simulink model "model_maglev"  (R2024a)
settings: Solver=VariableStepAuto  StartTime=0.0  StopTime=10.0  RelTol=1e-3
undefined symbols (not defined in the file): A, Cd, ci, fiP1, fiP2, g, ki, m, R, rho, v0, z0
settings Model: Creator=Bocchio  LastModifiedBy=Bocchio

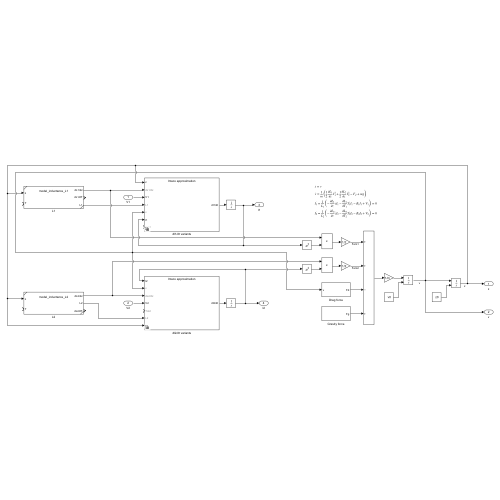
[thumbnail: Simulink's stored preview of the top-level diagram]
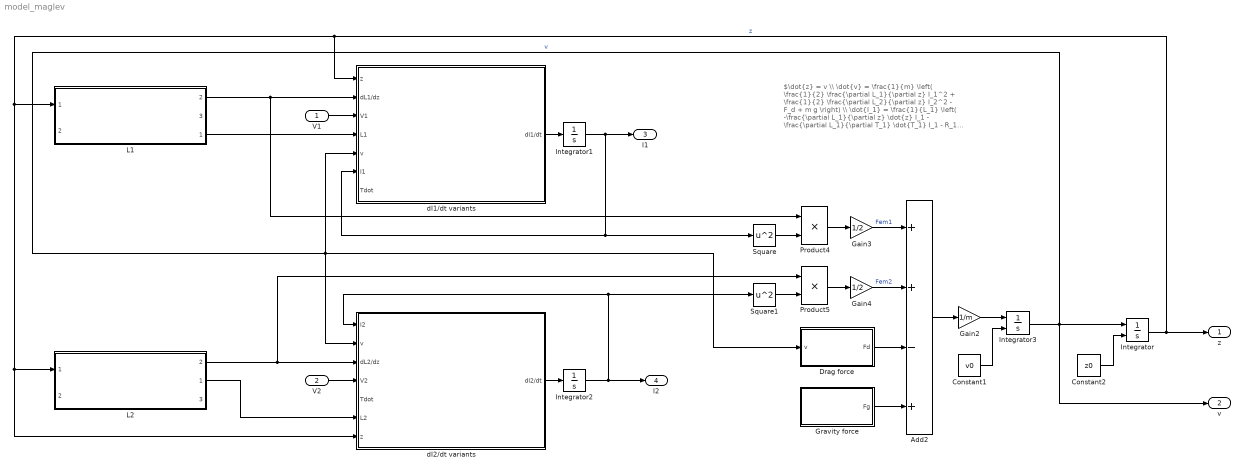
== system model_maglev ==
  note: $\dot{z} = v \\ \dot{v} = \frac{1}{m} \left( \frac{1}{2} \frac{\partial L_1}{\partial z} I_1^2 + \frac{1}{2} \frac{\partial L_2}{\partial z} I_2^2 - F_d + m g \right) \\ \dot{I_1} = \frac{1}{L_1} \left( -\frac{\partial L_1}{\partial z} \dot{z} I_1 - \frac{\partial L_1}{\partial T_1} \dot{T_1} I_1 - R_1 I_1 + V_1 \right) = 0 \\ \dot{I_2} = \frac{1}{L_2} \left( -\frac{\partial L_2}{\partial z} \dot{z} I_2 - \frac{\partial L_2}{\partial T_2} \dot{T_2} I_2 - R_2 I_2 + V_2 \right) = 0$
  V1 : Inport
  V2 : Inport  Port=2
  Add2 : Sum  Inputs=++-+
  Constant1 : Constant  Value=v0
  Constant2 : Constant  Value=z0
  Drag force : Subsystem
  Gain2 : Gain  Gain=1/m
  Gain3 : Gain  Gain=1/2
  Gain4 : Gain  Gain=1/2
  Gravity force : Subsystem
  Integrator : Integrator  InitialConditionSource=external
  Integrator1 : Integrator
  Integrator2 : Integrator
  Integrator3 : Integrator  InitialConditionSource=external
  L1 : Subsystem  ReferencedSubsystem=model_inductance_L1
      settings: PortSchema="{\"entries\":[{\"content\":{\"sides\":[{\"content\":{\"connectorIds\":[\"In1\",\"In2\"]},\"type\":\"ConnectorPlacement.EquallySpacedRectSide\",\"uuid\":\"7eb98e79-1222-4180-ad1b-16015b2454e9\"},{\"content\":{\"connectorIds\":[\"Out2\",\"Out3\",\"Out1\"],\"side\":\"RIGHT\"},\"type\":\"ConnectorPlacement.EquallySpacedRectSide\",\"uuid\":\"ce7d8014-b2ab-4313-9aa1-af3c9ff32da8\"},{\"content\":{\"side\":\"TOP\"},\"type\":\"ConnectorPlacement.EquallySpacedRectSide\",\"uuid\":\"6bd72466-ab25-4d86-adcd-22d1f13a01c9\"}]},\"type\":\"ConnectorPlacement.EquallySpacedConnector\",\"uuid\":\"baaaeab3-d8cd-49b4-9261-57480d9625ca\"}],\"packageUris\":[\"http://schema.mathworks.com/mf0/Connector/R2020b\"],\"version\":\"1.0\"}"
  L2 : Subsystem  ReferencedSubsystem=model_inductance_L2
      settings: PortSchema="{\"entries\":[{\"content\":{\"sides\":[{\"content\":{\"connectorIds\":[\"In1\",\"In2\"]},\"type\":\"ConnectorPlacement.EquallySpacedRectSide\",\"uuid\":\"1e02beb1-2eb2-4867-b71d-7851c60b3d68\"},{\"content\":{\"connectorIds\":[\"Out2\",\"Out1\",\"Out3\"],\"side\":\"RIGHT\"},\"type\":\"ConnectorPlacement.EquallySpacedRectSide\",\"uuid\":\"344f63f1-a805-4e14-b05f-49edc1fe2f4c\"},{\"content\":{\"side\":\"TOP\"},\"type\":\"ConnectorPlacement.EquallySpacedRectSide\",\"uuid\":\"d9945970-5ec1-4fd6-a2b8-3934b3c2782b\"}]},\"type\":\"ConnectorPlacement.EquallySpacedConnector\",\"uuid\":\"87b64261-f50a-433f-9b00-8a3b81ee7894\"}],\"packageUris\":[\"http://schema.mathworks.com/mf0/Connector/R2020b\"],\"version\":\"1.0\"}"
  Product4 : Product
  Product5 : Product
  Square : Math  Operator=square
  Square1 : Math  Operator=square
  dI1/dt variants : Subsystem  Variant=on  VariantControlMode=label  LabelModeActiveChoice=false
  dI2/dt variants : Subsystem  Variant=on  VariantControlMode=label  LabelModeActiveChoice=false
  z : Outport
  v : Outport  Port=2
  I1 : Outport  Port=3
  I2 : Outport  Port=4
  wires:
  Integrator/1 -> z/1, dI2/dt variants/7(z), L2/1, L1/1, dI1/dt variants/1(z)  "z"
  L1/1 -> dI1/dt variants/4(L1)
  Gain3/1 -> Add2/1  "Fem1"
  L2/1 -> dI2/dt variants/6(L2)
  dI1/dt variants/1(dI1/dt) -> Integrator1/1
  Gain4/1 -> Add2/2  "Fem2"
  Square/1 -> Product4/2
  Square1/1 -> Product5/2
  Integrator1/1 -> Square/1, dI1/dt variants/6(I1), I1/1
  Add2/1 -> Gain2/1
  Product4/1 -> Gain3/1
  Product5/1 -> Gain4/1
  Integrator3/1 -> v/1, Drag force/1(v), dI2/dt variants/2(v), dI1/dt variants/5(v), Integrator/1  "v"
  Integrator2/1 -> I2/1, Square1/1, dI2/dt variants/1(I2)
  V1/1 -> dI1/dt variants/3(V1)
  Drag force/1(Fd) -> Add2/3
  Gain2/1 -> Integrator3/1
  Constant1/1 -> Integrator3/2
  Constant2/1 -> Integrator/2
  Gravity force/1(Fg) -> Add2/4
  L1/2 -> Product4/1, dI1/dt variants/2(dL1/dz)
  dI2/dt variants/1(dI2/dt) -> Integrator2/1
  V2/1 -> dI2/dt variants/4(V2)
  L2/2 -> Product5/1, dI2/dt variants/3(dL2/dz)

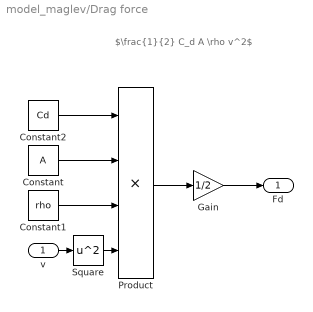
== system model_maglev/Drag force ==
  note: $\frac{1}{2} C_d A \rho v^2$
  v : Inport
  Constant : Constant  Value=A
  Constant1 : Constant  Value=rho
  Constant2 : Constant  Value=Cd
  Gain : Gain  Gain=1/2
  Product : Product  Inputs=4
  Square : Math  Operator=square
  Fd : Outport
  wires:
  Constant1/1 -> Product/3
  Constant/1 -> Product/2
  Constant2/1 -> Product/1
  Gain/1 -> Fd/1
  Product/1 -> Gain/1
  v/1 -> Square/1
  Square/1 -> Product/4

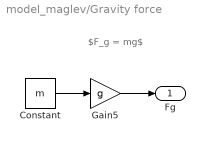
== system model_maglev/Gravity force ==
  note: $F_g = mg$
  Constant : Constant  Value=m
  Gain5 : Gain  Gain=g
  Fg : Outport
  wires:
  Gain5/1 -> Fg/1
  Constant/1 -> Gain5/1

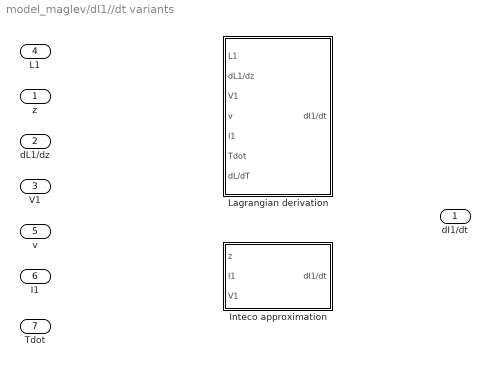
== system model_maglev/dI1//dt variants ==
  z : Inport
  dL1/dz : Inport  Port=2
  V1 : Inport  Port=3
  L1 : Inport  Port=4
  v : Inport  Port=5
  I1 : Inport  Port=6
  Tdot : Inport  Port=7
  Inteco approximation : Subsystem  VariantControl=false
  Lagrangian derivation : Subsystem  VariantControl=true
  dI1/dt : Outport

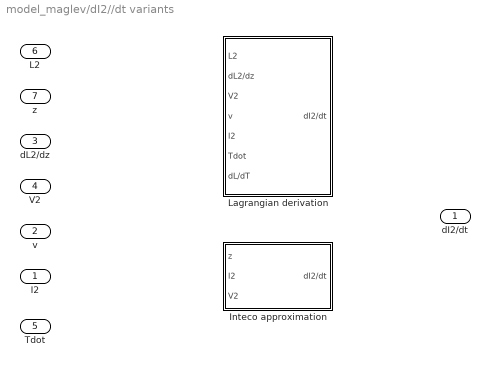
== system model_maglev/dI2//dt variants ==
  I2 : Inport
  v : Inport  Port=2
  dL2/dz : Inport  Port=3
  V2 : Inport  Port=4
  Tdot : Inport  Port=5
  L2 : Inport  Port=6
  z : Inport  Port=7
  Inteco approximation : Subsystem  VariantControl=false
  Lagrangian derivation : Subsystem  VariantControl=true
  dI2/dt : Outport

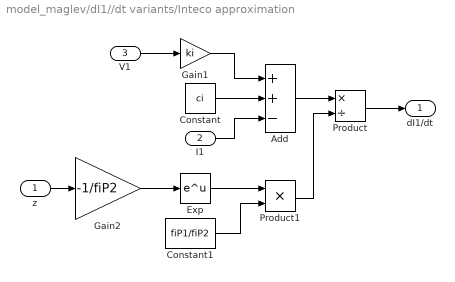
== system model_maglev/dI1//dt variants/Inteco approximation ==
  z : Inport
  I1 : Inport  Port=2
  V1 : Inport  Port=3
  Add : Sum  Inputs=++-
  Constant : Constant  Value=ci
  Constant1 : Constant  Value=fiP1/fiP2
  Exp : Math
  Gain1 : Gain  Gain=ki
  Gain2 : Gain  Gain=-1/fiP2
  Product : Product  Inputs=*/
  Product1 : Product
  dI1/dt : Outport
  wires:
  z/1 -> Gain2/1
  Gain1/1 -> Add/1
  I1/1 -> Add/3
  V1/1 -> Gain1/1
  Constant1/1 -> Product1/2
  Exp/1 -> Product1/1
  Constant/1 -> Add/2
  Gain2/1 -> Exp/1
  Add/1 -> Product/1
  Product1/1 -> Product/2
  Product/1 -> dI1/dt/1

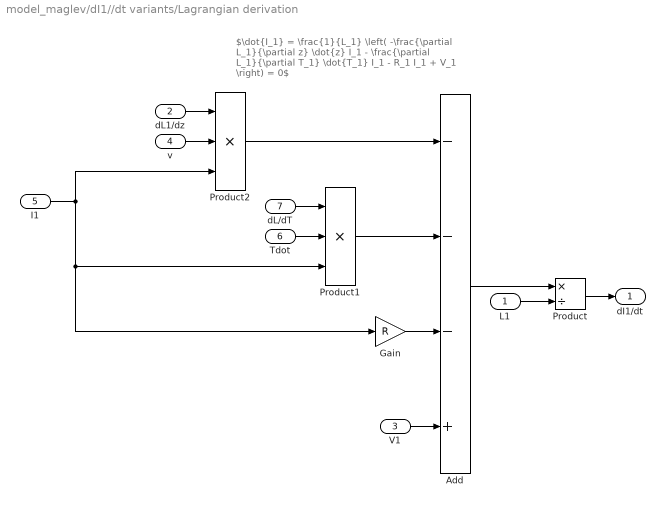
== system model_maglev/dI1//dt variants/Lagrangian derivation ==
  note: $\dot{I_1} = \frac{1}{L_1} \left( -\frac{\partial L_1}{\partial z} \dot{z} I_1 - \frac{\partial L_1}{\partial T_1} \dot{T_1} I_1 - R_1 I_1 + V_1 \right) = 0$
  L1 : Inport
  dL1/dz : Inport  Port=2
  V1 : Inport  Port=3
  v : Inport  Port=4
  I1 : Inport  Port=5
  Tdot : Inport  Port=6
  dL/dT : Inport  Port=7
  Add : Sum  Inputs=---+
  Gain : Gain  Gain=R
  Product : Product  Inputs=*/
  Product1 : Product  Inputs=3
  Product2 : Product  Inputs=3
  dI1/dt : Outport
  wires:
  Add/1 -> Product/1
  V1/1 -> Add/4
  Product2/1 -> Add/1
  Gain/1 -> Add/3
  Product/1 -> dI1/dt/1
  L1/1 -> Product/2
  v/1 -> Product2/2
  dL1/dz/1 -> Product2/1
  I1/1 -> Product2/3, Gain/1, Product1/3
  Product1/1 -> Add/2
  dL/dT/1 -> Product1/1
  Tdot/1 -> Product1/2

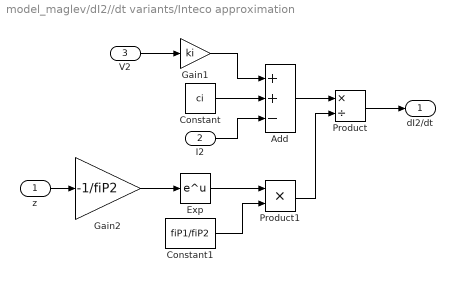
== system model_maglev/dI2//dt variants/Inteco approximation ==
  z : Inport
  I2 : Inport  Port=2
  V2 : Inport  Port=3
  Add : Sum  Inputs=++-
  Constant : Constant  Value=ci
  Constant1 : Constant  Value=fiP1/fiP2
  Exp : Math
  Gain1 : Gain  Gain=ki
  Gain2 : Gain  Gain=-1/fiP2
  Product : Product  Inputs=*/
  Product1 : Product
  dI2/dt : Outport
  wires:
  Product/1 -> dI2/dt/1
  Product1/1 -> Product/2
  Add/1 -> Product/1
  Gain2/1 -> Exp/1
  Constant/1 -> Add/2
  Exp/1 -> Product1/1
  Constant1/1 -> Product1/2
  V2/1 -> Gain1/1
  I2/1 -> Add/3
  Gain1/1 -> Add/1
  z/1 -> Gain2/1

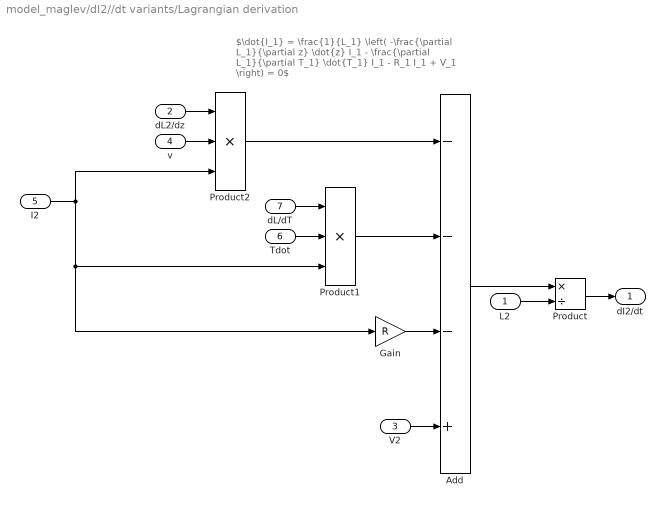
== system model_maglev/dI2//dt variants/Lagrangian derivation ==
  note: $\dot{I_1} = \frac{1}{L_1} \left( -\frac{\partial L_1}{\partial z} \dot{z} I_1 - \frac{\partial L_1}{\partial T_1} \dot{T_1} I_1 - R_1 I_1 + V_1 \right) = 0$
  L2 : Inport
  dL2/dz : Inport  Port=2
  V2 : Inport  Port=3
  v : Inport  Port=4
  I2 : Inport  Port=5
  Tdot : Inport  Port=6
  dL/dT : Inport  Port=7
  Add : Sum  Inputs=---+
  Gain : Gain  Gain=R
  Product : Product  Inputs=*/
  Product1 : Product  Inputs=3
  Product2 : Product  Inputs=3
  dI2/dt : Outport
  wires:
  Tdot/1 -> Product1/2
  dL/dT/1 -> Product1/1
  Product1/1 -> Add/2
  I2/1 -> Product1/3, Gain/1, Product2/3
  dL2/dz/1 -> Product2/1
  v/1 -> Product2/2
  L2/1 -> Product/2
  Product/1 -> dI2/dt/1
  Gain/1 -> Add/3
  Product2/1 -> Add/1
  V2/1 -> Add/4
  Add/1 -> Product/1
